simulink model "tiltrotor_model3"  (R2023a)
settings: Solver=FixedStepAuto  StartTime=0.0  StopTime=25  RelTol=1e-3
values from neighbouring files (symbols this model uses):
  delay_tilt = 0.004    [simulation_parameters.m]
  g = 9.81    [LQR_controller_pitching.m]    (also in MPC_controller_pitching.m; MPC_vs_LQR.m; simulation_parameters.m)
  I = diag([0.018 0.035 0.051])    [simulation_parameters.m]
  initial = [0 0 0 0 0 0]'    [simulation_parameters.m]
  kf = 65    [simulation_parameters.m]
  Lh = 0.2    [simulation_parameters.m]
  Lv = 0.2    [simulation_parameters.m]
  m = 1.12    [LQR_controller_pitching.m]    (also in MPC_vs_LQR.m = size(Bd,2); simulation_parameters.m)
  pitch_D = 0.4    [controller_parameters.m]    (also in controller_parameters_model_3_and_4.m; controller_parameters_model_5_and_6.m = 0)
  pitch_I = 0    [controller_parameters.m]    (also in controller_parameters_model_3_and_4.m; controller_parameters_model_5_and_6.m)
  pitch_P = 1.4    [controller_parameters.m]    (also in controller_parameters_model_3_and_4.m; controller_parameters_model_5_and_6.m = 10)
  reference = [0 0 1 0 50 45]'    [simulation_parameters.m]
  roll_D = 0.3    [controller_parameters.m]    (also in controller_parameters_model_3_and_4.m; controller_parameters_model_5_and_6.m = 1)
  roll_I = 0    [controller_parameters.m]    (also in controller_parameters_model_3_and_4.m; controller_parameters_model_5_and_6.m)
  roll_P = 1.5    [controller_parameters.m]    (also in controller_parameters_model_3_and_4.m; controller_parameters_model_5_and_6.m = 8)
  s_r = [1 1 1 1 1 1]    [simulation_parameters.m]
  Tmax = 4    [simulation_parameters.m]
  toll = 1e-12    [simulation_parameters.m]
  vx_D = 0    [controller_parameters.m]    (also in controller_parameters_model_3_and_4.m)
  vx_I = 0    [controller_parameters.m]    (also in controller_parameters_model_3_and_4.m)
  vx_P = 5    [controller_parameters.m]    (also in controller_parameters_model_3_and_4.m)
  vy_D = 0    [controller_parameters.m]    (also in controller_parameters_model_3_and_4.m; controller_parameters_model_5_and_6.m)
  vy_I = 0    [controller_parameters.m]    (also in controller_parameters_model_3_and_4.m; controller_parameters_model_5_and_6.m)
  vy_P = 5    [controller_parameters.m]    (also in controller_parameters_model_3_and_4.m; controller_parameters_model_5_and_6.m = 12)
  vz_D = 0    [controller_parameters.m]    (also in controller_parameters_model_3_and_4.m)
  vz_I = 1.5    [controller_parameters.m]    (also in controller_parameters_model_3_and_4.m = 0)
  vz_P = 9    [controller_parameters.m]    (also in controller_parameters_model_3_and_4.m)
  x_D = 0.7    [controller_parameters.m]    (also in controller_parameters_model_3_and_4.m; controller_parameters_model_5_and_6.m = 0)
  x_I = 0    [controller_parameters.m]    (also in controller_parameters_model_3_and_4.m; controller_parameters_model_5_and_6.m)
  x_P = 1.8    [controller_parameters.m]    (also in controller_parameters_model_3_and_4.m; controller_parameters_model_5_and_6.m = 1.5)
  y_D = 0.7    [controller_parameters.m]    (also in controller_parameters_model_3_and_4.m; controller_parameters_model_5_and_6.m = 0.3)
  y_I = 0    [controller_parameters.m]    (also in controller_parameters_model_3_and_4.m; controller_parameters_model_5_and_6.m)
  y_P = 1.8    [controller_parameters.m]    (also in controller_parameters_model_3_and_4.m; controller_parameters_model_5_and_6.m = 1.5)
  yaw_D = 0.5    [controller_parameters.m]    (also in controller_parameters_model_3_and_4.m = 0.3; controller_parameters_model_5_and_6.m = 0)
  yaw_I = 0    [controller_parameters.m]    (also in controller_parameters_model_3_and_4.m; controller_parameters_model_5_and_6.m)
  yaw_P = 1    [controller_parameters.m]    (also in controller_parameters_model_3_and_4.m; controller_parameters_model_5_and_6.m = 1.5)
  z_D = 0    [controller_parameters.m]    (also in controller_parameters_model_3_and_4.m; controller_parameters_model_5_and_6.m)
  z_I = 0    [controller_parameters.m]    (also in controller_parameters_model_3_and_4.m; controller_parameters_model_5_and_6.m)
  z_P = 3    [controller_parameters.m]    (also in controller_parameters_model_3_and_4.m; controller_parameters_model_5_and_6.m = 2.5)
libraries: slpidlib x9, simulink x6, simulink_extras x2, matrix_library x1
(part 2 of 2)

== matlab function tiltrotor_model3/Control allocation/MATLAB Function1 ==
  data: eta input; D output; Lv input; Lh input; kf input
function D = fcn(eta, Lv, Lh, kf)

kf = 1/kf;

D = 0.25*[1, -1/kf * sin(eta) - 1/Lh * cos(eta), - 1/Lv / cos(eta), -1/kf * cos(eta) + 1/Lh * sin(eta);
    1, 1/kf * sin(eta) + 1/Lh * cos(eta), - 1/Lv / cos(eta), 1/kf * cos(eta) - 1/Lh * sin(eta);
    1, -1/kf * sin(eta) + 1/Lh * cos(eta), 1/Lv / cos(eta), -1/kf * cos(eta) - 1/Lh * sin(eta);
    1, 1/kf * sin(eta) - 1/Lh * cos(eta), 1/Lv / cos(eta), 1/kf * cos(eta) + 1/Lh * sin(eta)];

== matlab function tiltrotor_model3/UAV/Dynamics of phi/MATLAB Function1 ==
  data: phi input; Q output
function Q = fcn(phi)

roll = phi(1);
pitch = phi(2);

Q = euler_to_body_angvel(roll, pitch);

== matlab function tiltrotor_model3/UAV/MATLAB Function ==
  data: Rx output; Ry output; Rz output; phi input
function [Rx, Ry, Rz]  = fcn(phi)

roll = phi(1);
pitch = phi(2);
yaw = phi(3);

[Rx, Ry, Rz] = rotation_matrices(roll, pitch, yaw);
